simulink model "plc"  (R2023a)
settings: Solver=VariableStepAuto  StartTime=0.0  StopTime=inf  RelTol=1e-3
values from neighbouring files (symbols this model uses):
  a1 = 0.45    [init.m]
  A1 = 154    [init.m]
  a2 = 0.25    [init.m]
  A3 = 154    [init.m]
  g = 980.665    [init.m]
  H1_max = 100    [init.m]
  Q1_max = 100    [init.m]
  Q3_max = 10    [init.m]
  s12 = 0.5    [init.m]
  s23 = s12    (= 0.5)    [init.m]
libraries: dspnetwork x9
settings Model: Creator=Dottorandi  LastModifiedBy=mattia
settings SolverCC: AlgebraicLoopSolver=TrustRegion
settings DataIOCC: ReturnWorkspaceOutputs=off
settings DebuggingCC: UnconnectedInputMsg=warning  UnconnectedOutputMsg=warning  UnconnectedLineMsg=warning  ArithmeticOperatorsInVariantConditions=warning
settings ModelReferenceCC: EnableRefExpFcnMdlSchedulingChecks=on
settings SFSimCC: SimUseLocalCustomCode=off  CustomCodeUndefinedFunction=UseInterfaceOnly
settings RTWCC: RTWUseLocalCustomCode=off  DLArmComputeVersion=19.05

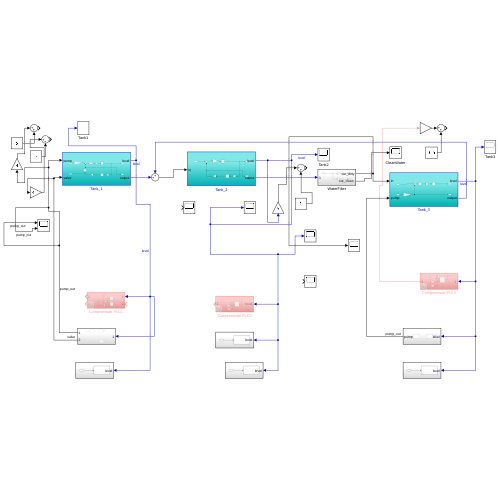
[thumbnail: Simulink's stored preview of the top-level diagram]
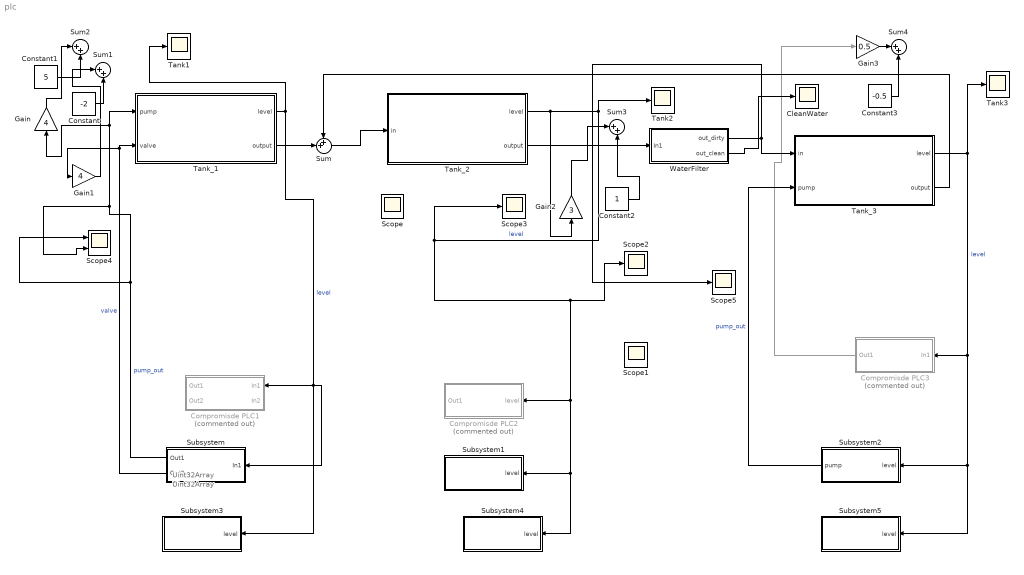
== system plc ==
  note: Uint32Array
  note: Uint32Array
  "CleanWater " : Scope
  Compromisde PLC1 : Subsystem  Commented=on
  Compromisde PLC2 : Subsystem  Commented=on
  Compromisde PLC3 : Subsystem  Commented=on
  Constant : Constant  Value=-2
  Constant1 : Constant  Value=5
  Constant2 : Constant
  Constant3 : Constant  Value=-0.5
  Gain : Gain  Gain=4
  Gain1 : Gain  Gain=4
  Gain2 : Gain  Gain=3
  Gain3 : Gain  Gain=0.5
  Scope{,1..3,5} (5 alike) : Scope
  Scope4 : Scope  NumInputPorts=2
  Subsystem : Subsystem
  Subsystem1 : Subsystem
  Subsystem2 : Subsystem
  Subsystem3 : Subsystem
  Subsystem4 : Subsystem
  Subsystem5 : Subsystem
  Sum : Sum  Inputs=++|
  Sum{1..4} (4 alike) : Sum  Inputs=|++
  Tank1 : Scope
  Tank2 : Scope
  Tank3 : Scope
  Tank_1 : Subsystem
  Tank_2 : Subsystem
  Tank_3 : Subsystem
  WaterFilter : Subsystem
  wires:
  Tank_2/1(level) -> Gain2/1, Tank2/1, Subsystem4/1(level), Subsystem1/1(level), Compromisde PLC2/1(level), Scope2/1, Scope3/1  "level"
  Sum/1 -> Tank_2/1(in)
  Compromisde PLC3/1(Out1) -> Gain3/1
  Tank_1/1(level) -> Compromisde PLC1/1(In1), Subsystem/1(In1), Subsystem3/1(level), Tank1/1  "level"
  Tank_3/2(output) -> Sum/1
  WaterFilter/2("out_clean ") -> "CleanWater "/1
  Tank_1/2(output) -> Sum/2
  Subsystem/2(Out2) -> Gain1/1, Tank_1/2(valve)  "valve"
  Tank_2/2(output) -> WaterFilter/1(In1)
  Subsystem/1(Out1) -> Scope4/2, Tank_1/1(pump), Gain/1, Scope4/1  "pump_out"
  Constant/1 -> Sum1/2
  Constant1/1 -> Sum2/2
  Gain/1 -> Sum2/1
  Gain1/1 -> Sum1/1
  Constant2/1 -> Sum3/2
  Gain2/1 -> Sum3/1
  Constant3/1 -> Sum4/2
  Gain3/1 -> Sum4/1
  WaterFilter/1(out_dirty) -> Tank_3/1(in), Scope5/1
  Subsystem2/1(pump) -> Tank_3/2(pump)  "pump_out"
  Tank_3/1(level) -> Tank3/1, Compromisde PLC3/1(In1), Subsystem5/1(level), Subsystem2/1(level)  "level"

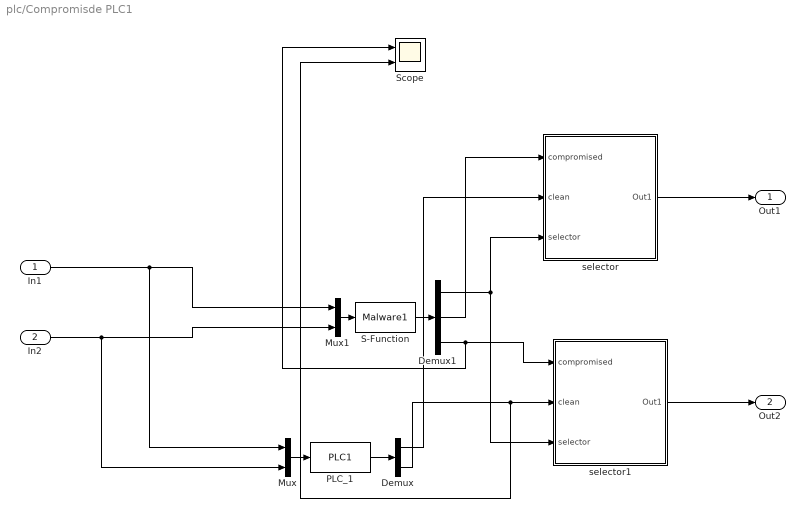
== system plc/Compromisde PLC1 ==
  In1 : Inport
  In2 : Inport  Port=2
  Demux : Demux  Outputs=2
  Demux1 : Demux  Outputs=3
  Mux : Mux  Inputs=2
  Mux1 : Mux  Inputs=2
  PLC_1 : S-Function  FunctionName=PLC1  SFunctionDeploymentMode=off  EnableBusSupport=off
  S-Function : S-Function  FunctionName=Malware1  SFunctionDeploymentMode=off  EnableBusSupport=off
  Scope : Scope  NumInputPorts=2
  selector : Subsystem
  selector1 : Subsystem
  Out1 : Outport  VectorParamsAs1DForOutWhenUnconnected=off
  Out2 : Outport  Port=2  VectorParamsAs1DForOutWhenUnconnected=off
  wires:
  Mux/1 -> PLC_1/1
  PLC_1/1 -> Demux/1
  Mux1/1 -> S-Function/1
  In1/1 -> Mux/1, Mux1/1
  In2/1 -> Mux/2, Mux1/2
  S-Function/1 -> Demux1/1
  Demux1/1 -> selector1/3(selector), selector/3(selector)
  Demux/1 -> selector/2(clean)
  Demux1/2 -> selector/1(compromised)
  Demux/2 -> Scope/2, selector1/2(clean)
  Demux1/3 -> selector1/1(compromised), Scope/1
  selector/1(Out1) -> Out1/1
  selector1/1(Out1) -> Out2/1

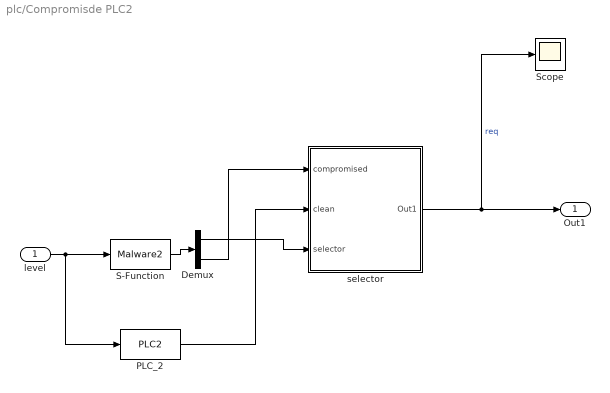
== system plc/Compromisde PLC2 ==
  level : Inport
  Demux : Demux  Outputs=2
  PLC_2 : S-Function  FunctionName=PLC2  SFunctionDeploymentMode=off  EnableBusSupport=off
  S-Function : S-Function  FunctionName=Malware2  SFunctionDeploymentMode=off  EnableBusSupport=off
  Scope : Scope
  selector : Subsystem
  Out1 : Outport  VectorParamsAs1DForOutWhenUnconnected=off
  wires:
  PLC_2/1 -> selector/2(clean)
  Demux/2 -> selector/1(compromised)
  selector/1(Out1) -> Scope/1, Out1/1  "req"
  Demux/1 -> selector/3(selector)
  S-Function/1 -> Demux/1
  level/1 -> PLC_2/1, S-Function/1

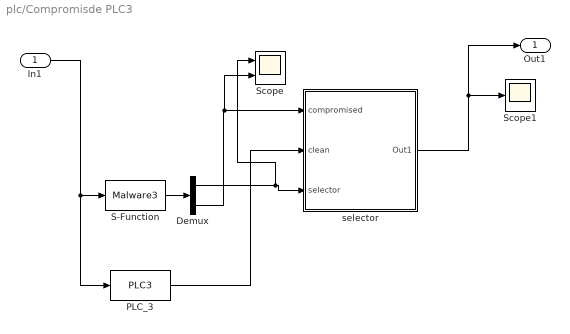
== system plc/Compromisde PLC3 ==
  In1 : Inport
  Demux : Demux  Outputs=2
  "PLC_3 " : S-Function  FunctionName=PLC3  SFunctionDeploymentMode=off  EnableBusSupport=off
  S-Function : S-Function  FunctionName=Malware3  SFunctionDeploymentMode=off  EnableBusSupport=off
  Scope : Scope  NumInputPorts=2
  Scope1 : Scope
  selector : Subsystem
  Out1 : Outport  VectorParamsAs1DForOutWhenUnconnected=off
  wires:
  In1/1 -> S-Function/1, "PLC_3 "/1
  "PLC_3 "/1 -> selector/2(clean)
  S-Function/1 -> Demux/1
  Demux/1 -> Scope/1, selector/3(selector)
  Demux/2 -> Scope/2, selector/1(compromised)
  selector/1(Out1) -> Out1/1, Scope1/1

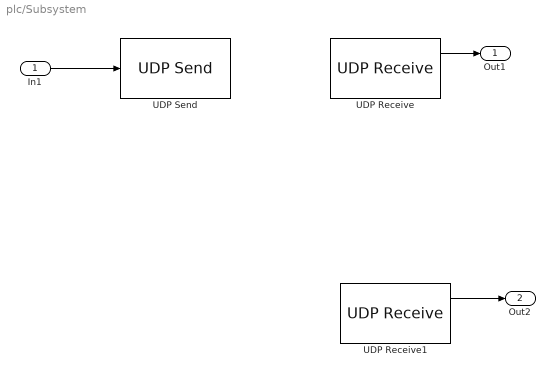
== system plc/Subsystem ==
  In1 : Inport
  UDP Receive : dspnetwork/UDP Receive  localURL='0.0.0.0'  localPort=10002  remoteURL='0.0.0.0'  remotePort=-1  recvBufferSize=2  dims=1  signalDatatype=uint16  isComplex=off  isVarSize=off  showBlockingTime=on  blockingTime=0  sampletime=1  blockPlatform=LINUX
  UDP Receive1 : dspnetwork/UDP Receive  localURL='0.0.0.0'  localPort=10003  remoteURL='0.0.0.0'  remotePort=-1  recvBufferSize=2  dims=1  signalDatatype=uint16  isComplex=off  isVarSize=off  showBlockingTime=on  blockingTime=0  sampletime=1  blockPlatform=LINUX
  UDP Send : dspnetwork/UDP Send  remoteURL='192.168.10.106'  remotePort=10001  localURL='255.255.255.255'  localPortSource=Automatically determine  localPort=-1  sendBufferSize=8192  sampletime=-1  blockPlatform=LINUX  separateLengthPort=0
  Out1 : Outport  VectorParamsAs1DForOutWhenUnconnected=off
  Out2 : Outport  Port=2  VectorParamsAs1DForOutWhenUnconnected=off
  wires:
  In1/1 -> UDP Send/1
  UDP Receive/1 -> Out1/1
  UDP Receive1/1 -> Out2/1

== system plc/Subsystem1 ==
  level : Inport
  UDP Send : dspnetwork/UDP Send  remoteURL='192.168.10.107'  remotePort=10004  localURL='255.255.255.255'  localPortSource=Automatically determine  localPort=-1  sendBufferSize=8192  sampletime=-1  blockPlatform=LINUX  separateLengthPort=0
  wires:
  level/1 -> UDP Send/1

== system plc/Subsystem2 ==
  level : Inport
  UDP Receive : dspnetwork/UDP Receive  localURL='0.0.0.0'  localPort=10006  remoteURL='0.0.0.0'  remotePort=-1  recvBufferSize=2  dims=1  signalDatatype=uint16  isComplex=off  isVarSize=off  showBlockingTime=on  blockingTime=0  sampletime=1  blockPlatform=LINUX
  UDP Send : dspnetwork/UDP Send  remoteURL='192.168.10.108'  remotePort=10005  localURL='255.255.255.255'  localPortSource=Automatically determine  localPort=-1  sendBufferSize=8192  sampletime=-1  blockPlatform=LINUX  separateLengthPort=0
  pump : Outport  VectorParamsAs1DForOutWhenUnconnected=off
  wires:
  level/1 -> UDP Send/1
  UDP Receive/1 -> pump/1

== system plc/Subsystem3 ==
  level : Inport
  UDP Send : dspnetwork/UDP Send  remoteURL='localhost'  remotePort=10007  localURL='255.255.255.255'  localPortSource=Automatically determine  localPort=-1  sendBufferSize=8192  sampletime=-1  blockPlatform=LINUX  separateLengthPort=0
  wires:
  level/1 -> UDP Send/1

== system plc/Subsystem4 ==
  level : Inport
  UDP Send : dspnetwork/UDP Send  remoteURL='localhost'  remotePort=10008  localURL='255.255.255.255'  localPortSource=Automatically determine  localPort=-1  sendBufferSize=8192  sampletime=-1  blockPlatform=LINUX  separateLengthPort=0
  wires:
  level/1 -> UDP Send/1

== system plc/Subsystem5 ==
  level : Inport
  UDP Send : dspnetwork/UDP Send  remoteURL='localhost'  remotePort=10009  localURL='255.255.255.255'  localPortSource=Automatically determine  localPort=-1  sendBufferSize=8192  sampletime=-1  blockPlatform=LINUX  separateLengthPort=0
  wires:
  level/1 -> UDP Send/1

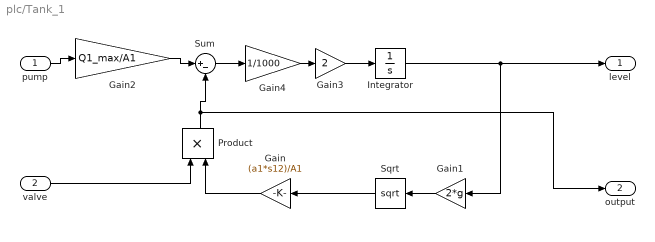
== system plc/Tank_1 ==
  pump : Inport
  valve : Inport  Port=2
  Gain : Gain  Gain=(a1*s12)/A1
  Gain1 : Gain  Gain=2*g
  Gain2 : Gain  Gain=Q1_max/A1
  Gain3 : Gain  Gain=2
  Gain4 : Gain  Gain=1/1000
  Integrator : Integrator  InitialCondition=0.11*H1_max  LimitOutput=on  UpperSaturationLimit=100  LowerSaturationLimit=0
  Product : Product
  Sqrt : Sqrt
  Sum : Sum  Inputs=|+-
  level : Outport  VectorParamsAs1DForOutWhenUnconnected=off
  output : Outport  Port=2  VectorParamsAs1DForOutWhenUnconnected=off
  wires:
  pump/1 -> Gain2/1
  Integrator/1 -> Gain1/1, level/1
  Sum/1 -> Gain4/1
  Gain/1 -> Product/2
  Sqrt/1 -> Gain/1
  Gain1/1 -> Sqrt/1
  valve/1 -> Product/1
  Product/1 -> output/1, Sum/2
  Gain2/1 -> Sum/1
  Gain3/1 -> Integrator/1
  Gain4/1 -> Gain3/1

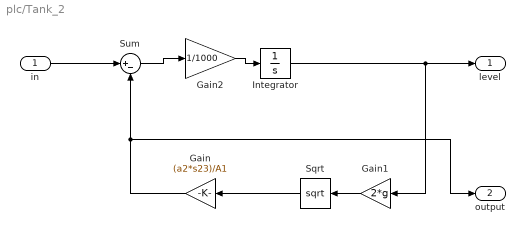
== system plc/Tank_2 ==
  in : Inport
  Gain : Gain  Gain=(a2*s23)/A1
  Gain1 : Gain  Gain=2*g
  Gain2 : Gain  Gain=1/1000
  Integrator : Integrator  InitialCondition=0.11*H1_max  LimitOutput=on  UpperSaturationLimit=30  LowerSaturationLimit=0
  Sqrt : Sqrt
  Sum : Sum  Inputs=|+-
  level : Outport  VectorParamsAs1DForOutWhenUnconnected=off
  output : Outport  Port=2  VectorParamsAs1DForOutWhenUnconnected=off
  wires:
  in/1 -> Sum/1
  Integrator/1 -> Gain1/1, level/1
  Sum/1 -> Gain2/1
  Sqrt/1 -> Gain/1
  Gain1/1 -> Sqrt/1
  Gain/1 -> output/1, Sum/2
  Gain2/1 -> Integrator/1

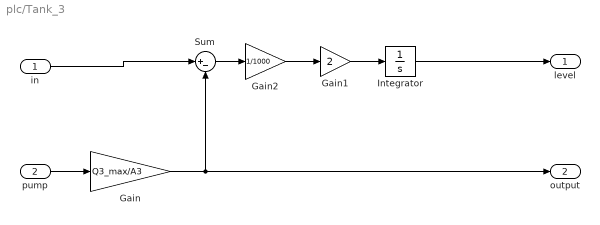
== system plc/Tank_3 ==
  in : Inport
  pump : Inport  Port=2
  Gain : Gain  Gain=Q3_max/A3
  Gain1 : Gain  Gain=2
  Gain2 : Gain  Gain=1/1000
  Integrator : Integrator  LimitOutput=on  LowerSaturationLimit=0
  Sum : Sum  Inputs=|+-
  level : Outport  VectorParamsAs1DForOutWhenUnconnected=off
  output : Outport  Port=2  VectorParamsAs1DForOutWhenUnconnected=off
  wires:
  Integrator/1 -> level/1
  Sum/1 -> Gain2/1
  pump/1 -> Gain/1
  in/1 -> Sum/1
  Gain/1 -> Sum/2, output/1
  Gain1/1 -> Integrator/1
  Gain2/1 -> Gain1/1

== system plc/WaterFilter ==
  In1 : Inport
  Gain : Gain  Gain=0.01
  Gain1 : Gain  Gain=0.99
  out_dirty : Outport  VectorParamsAs1DForOutWhenUnconnected=off
  "out_clean " : Outport  Port=2  VectorParamsAs1DForOutWhenUnconnected=off
  wires:
  In1/1 -> Gain1/1, Gain/1
  Gain/1 -> out_dirty/1
  Gain1/1 -> "out_clean "/1

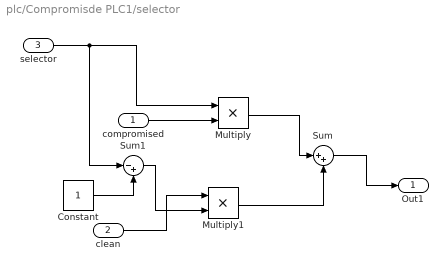
== system plc/Compromisde PLC1/selector ==
  compromised : Inport
  clean : Inport  Port=2
  selector : Inport  Port=3
  Constant : Constant
  Multiply : Product
  Multiply1 : Product
  Sum : Sum  Inputs=|++
  Sum1 : Sum  Inputs=|-+
  Out1 : Outport  VectorParamsAs1DForOutWhenUnconnected=off
  wires:
  compromised/1 -> Multiply/2
  clean/1 -> Multiply1/1
  selector/1 -> Sum1/1, Multiply/1
  Sum/1 -> Out1/1
  Multiply/1 -> Sum/1
  Multiply1/1 -> Sum/2
  Constant/1 -> Sum1/2
  Sum1/1 -> Multiply1/2

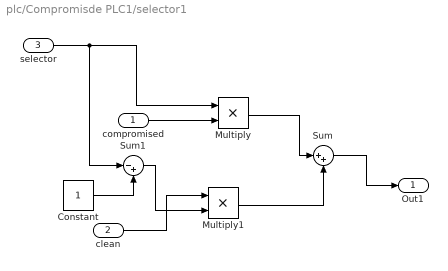
== system plc/Compromisde PLC1/selector1 ==
  compromised : Inport
  clean : Inport  Port=2
  selector : Inport  Port=3
  Constant : Constant
  Multiply : Product
  Multiply1 : Product
  Sum : Sum  Inputs=|++
  Sum1 : Sum  Inputs=|-+
  Out1 : Outport  VectorParamsAs1DForOutWhenUnconnected=off
  wires:
  compromised/1 -> Multiply/2
  clean/1 -> Multiply1/1
  selector/1 -> Sum1/1, Multiply/1
  Sum/1 -> Out1/1
  Multiply/1 -> Sum/1
  Multiply1/1 -> Sum/2
  Constant/1 -> Sum1/2
  Sum1/1 -> Multiply1/2

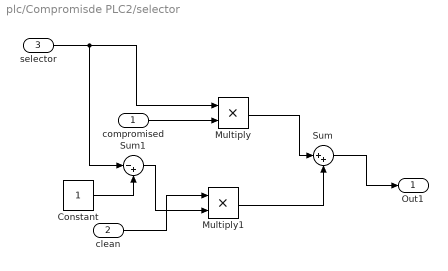
== system plc/Compromisde PLC2/selector ==
  compromised : Inport
  clean : Inport  Port=2
  selector : Inport  Port=3
  Constant : Constant
  Multiply : Product
  Multiply1 : Product
  Sum : Sum  Inputs=|++
  Sum1 : Sum  Inputs=|-+
  Out1 : Outport  VectorParamsAs1DForOutWhenUnconnected=off
  wires:
  compromised/1 -> Multiply/2
  clean/1 -> Multiply1/1
  selector/1 -> Sum1/1, Multiply/1
  Sum/1 -> Out1/1
  Multiply/1 -> Sum/1
  Multiply1/1 -> Sum/2
  Constant/1 -> Sum1/2
  Sum1/1 -> Multiply1/2

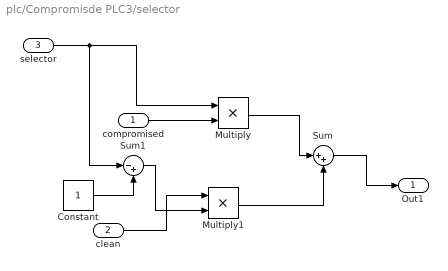
== system plc/Compromisde PLC3/selector ==
  compromised : Inport
  clean : Inport  Port=2
  selector : Inport  Port=3
  Constant : Constant
  Multiply : Product
  Multiply1 : Product
  Sum : Sum  Inputs=|++
  Sum1 : Sum  Inputs=|-+
  Out1 : Outport  VectorParamsAs1DForOutWhenUnconnected=off
  wires:
  compromised/1 -> Multiply/2
  clean/1 -> Multiply1/1
  selector/1 -> Sum1/1, Multiply/1
  Sum/1 -> Out1/1
  Multiply/1 -> Sum/1
  Multiply1/1 -> Sum/2
  Constant/1 -> Sum1/2
  Sum1/1 -> Multiply1/2
